simulink model "MatlabFunction"  (R2019b)
settings: Solver=VariableStepAuto  StartTime=0.0  StopTime=10.0  RelTol=1e-3
model workspace (MAT data in the model file):
  NITER = 0
  REF = 860
undefined symbols (not defined in the file): t_sim
libraries: legoev3lib x6, simulink x1
settings Model: Creator=alumnopr18  LastModifiedBy=alumnopr18

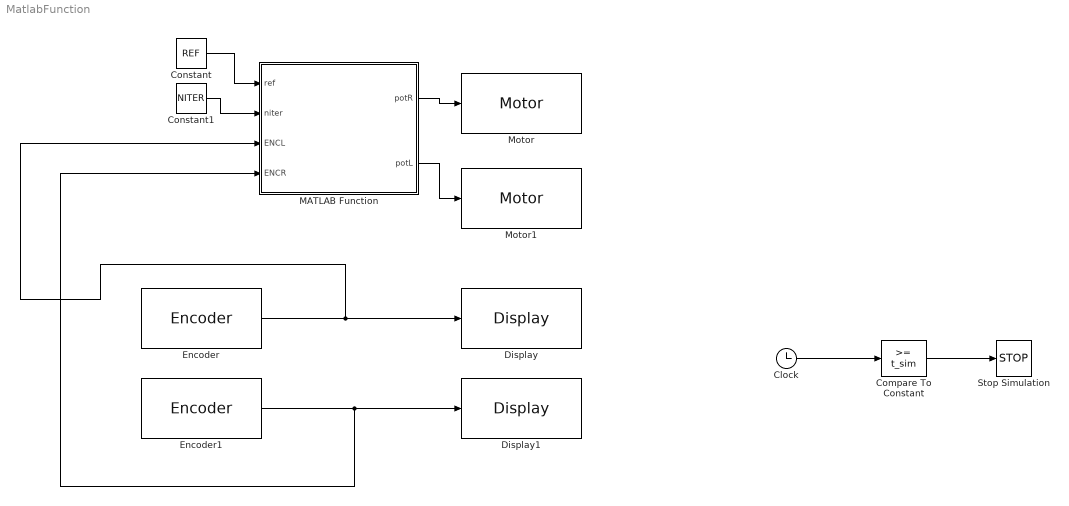
== system MatlabFunction ==
  Clock : Clock
  Compare To Constant : simulink/Logic and Bit Operations/Compare To Constant  relop=>=  const=t_sim  OutDataTypeStr=boolean
  Constant : Constant  Value=REF
  Constant1 : Constant  Value=NITER
  Display : legoev3lib/Display  slcdLine=1  slcdFormat=Decimal
      settings: SourceProductName=Simulink Support Package for LEGO MINDSTORMS EV3 Hardware  SourceProductBaseCode=LEGOEV3
  Display1 : legoev3lib/Display  slcdLine=2  slcdFormat=Decimal
      settings: SourceProductName=Simulink Support Package for LEGO MINDSTORMS EV3 Hardware  SourceProductBaseCode=LEGOEV3
  Encoder : legoev3lib/Encoder  portNumber=B  opMode=No reset  sampleTime=0.1
      settings: SourceProductName=Simulink Support Package for LEGO MINDSTORMS EV3 Hardware  SourceProductBaseCode=LEGOEV3
  Encoder1 : legoev3lib/Encoder  portNumber=C  opMode=No reset  sampleTime=0.1
      settings: SourceProductName=Simulink Support Package for LEGO MINDSTORMS EV3 Hardware  SourceProductBaseCode=LEGOEV3
  MATLAB Function : MATLAB Function  TreatAsAtomicUnit=on
  Motor : legoev3lib/Motor  sportNumber=B  sstopAction=Brake
  Motor1 : legoev3lib/Motor  sportNumber=C  sstopAction=Brake
  Stop Simulation : Stop
  wires:
  Compare To Constant/1 -> Stop Simulation/1
  Clock/1 -> Compare To Constant/1
  Encoder/1 -> MATLAB Function/3(ENCL), Display/1
  Encoder1/1 -> MATLAB Function/4(ENCR), Display1/1
  Constant/1 -> MATLAB Function/1(ref)
  Constant1/1 -> MATLAB Function/2(niter)
  MATLAB Function/1(potR) -> Motor/1
  MATLAB Function/2(potL) -> Motor1/1

== matlab function MatlabFunction/MATLAB Function ==
  data: ref input; potR output; niter input; ENCL input; ENCR input; potL output
function [potR,potL] = fcn(ref,niter,ENCL,ENCR)

persistent iter;

if(isempty(iter))
  iter = 0;
end

if(iter <= niter)
    if(ENCL >= 100)
        ENCL = int32(100)
    end
    if(ENCR <= -100)
        ENCR = int32(-100)
    end
    potR = int32(ref - ENCR)
    potL = int32(ref - ENCL)
    
end

iter = iter + 1; 
end
